simulink subsystem "robot_mc"  (R2021b)
settings: Solver=VariableStepAuto  StartTime=0.0  StopTime=10.0  RelTol=1e-3
settings Model: Creator=marco  LastModifiedBy=angelo

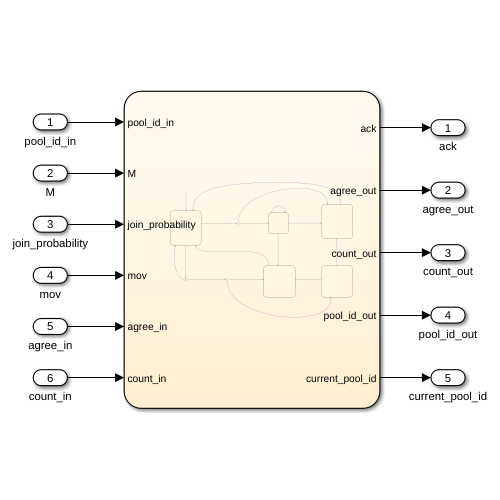
[thumbnail: Simulink's stored preview of the top-level diagram]
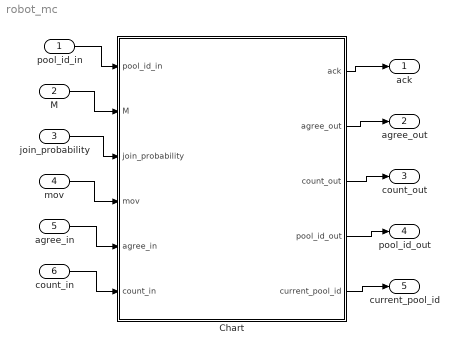
== system robot_mc ==
  pool_id_in : Inport
  M : Inport  Port=2
  join_probability : Inport  Port=3
  mov : Inport  Port=4
  agree_in : Inport  Port=5
  count_in : Inport  Port=6
  Chart : Stateflow chart  TreatAsAtomicUnit=on
  ack : Outport
  agree_out : Outport  Port=2
  count_out : Outport  Port=3
  pool_id_out : Outport  Port=4
  current_pool_id : Outport  Port=5
  wires:
  pool_id_in/1 -> Chart/1(pool_id_in)
  M/1 -> Chart/2(M)
  join_probability/1 -> Chart/3(join_probability)
  Chart/1(ack) -> ack/1
  Chart/2(agree_out) -> agree_out/1
  Chart/3(count_out) -> count_out/1
  mov/1 -> Chart/4(mov)
  agree_in/1 -> Chart/5(agree_in)
  count_in/1 -> Chart/6(count_in)
  Chart/4(pool_id_out) -> pool_id_out/1
  Chart/5(current_pool_id) -> current_pool_id/1

== stateflow chart robot_mc/Chart ==
  state Processing
    du: pool_id_out = 0;
    state Abort
      entry:
      if (~is_coord)
      agree_out = -1;
      else
      ack = -1;
      end
      exit:
      agree_out = 0;
      ack = 0;
    state Coordination
      during:
      count_out = 0;
      agree_out = 0;
    state CommonAction
      entry:
      current_pool_id = pool_id;
      during:
      agree_out = agree_in;
      ack = 0;
      count_out = count_in;
      pool_id_out = pool_id_in;
      exit:
      current_pool_id = 0;
      pool_id_out = pool_id_in;
      count_out = count_in;
      % agree_out = 0;
      agree_out = agree_in;
    state AgreeWait
      entry:
      count_out = count_in + 1;
      during:
      count_out = 0;
    Coordination -> Coordination [order 1] : % pool failed
        | [(count_in > 0) & (pool_id == pool_id_in)]
        | {agree_out = -1;}
    Coordination -> Abort [order 3] : % failure
        | [agree_in == -1]
    Coordination -> CommonAction [order 2] : % success
        | [agree_in == 1]
        | {ack = 1;}
    AgreeWait -> Abort [order 2] : % failure
        | [agree_in == -1]
    AgreeWait -> CommonAction [order 1] : % commit
        | [agree_in == 1]
        | {agree_out = 1;}
  state MovWait
    entry:
    is_coord = 0;
    pool_id = 0;
    during:
    join = (join_probability > 0.5);
    count_out = 0;
    agree_out = agree_in;
    pool_id_out = 0;
  Abort -> MovWait
  (junction 99) -> Abort [order 2]
  (default) -> MovWait : {join = (join_probability > 0.5);}
  MovWait -> (junction 99) [order 1] : % request received
      | [mov & (count_in == 0)]
      | {is_coord = 1;
      |  pool_id = pool_id_in;}
  (junction 99) -> Coordination [order 1] : [join]
      | {count_out = 1;
      |  pool_id_out = pool_id_in;}
  (junction 105) -> MovWait [order 2] : {count_out = count_in;
      |  pool_id_out = pool_id_in;}
  MovWait -> (junction 105) [order 2] : % query to commit
      | [count_in > 0]
  CommonAction -> MovWait : after(2,sec)
  (junction 105) -> (junction 111) [order 1] : [join]
      | {pool_id = pool_id_in;}
  (junction 111) -> CommonAction [order 1] : % pool formed
      | [count_in+1 == M]
      | {agree_out = 1;}
  (junction 111) -> AgreeWait [order 2] : % agree
      | {pool_id_out = pool_id_in;}
  data: pool_id_in input; M input; join_probability input; join local; mov input; ack output =0; agree_in input; count_in input; agree_out output =0; count_out output =0; is_coord local =0; pool_id_out output; pool_id local =0; current_pool_id output =0
